simulink model "QUATERNIONS_control_law"  (R2022b)
settings: Solver=VariableStepAuto  StartTime=0.0  StopTime=10.0  RelTol=1e-3
undefined symbols (not defined in the file or in its folder): A_ATTITUDE_DET, K_d, Kp, W_e
settings Model: Creator=carlorichero  LastModifiedBy=carlorichero
settings OptimizationCC: ReuseModelBlockBuffer=on
settings RTWCC: GPUComputeCapability=5.0

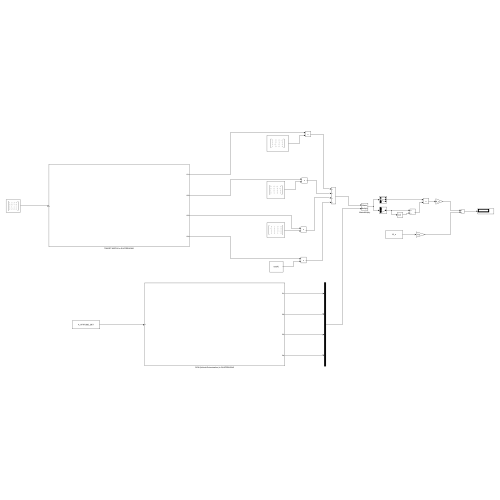
[thumbnail: Simulink's stored preview of the top-level diagram]
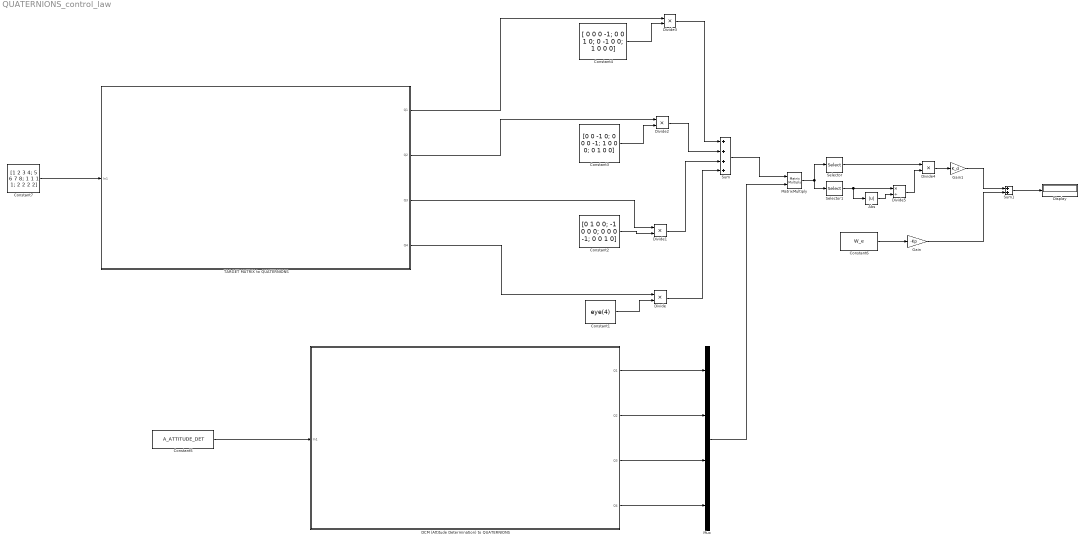
== system QUATERNIONS_control_law ==
  Abs : Abs  SaturateOnIntegerOverflow=off
  Constant1 : Constant  Value=eye(4)
  Constant2 : Constant  Value=[0 1 0 0; -1 0 0 0; 0 0 0 -1; 0 0 1 0]
  Constant3 : Constant  Value=[0 0 -1 0; 0 0 0 -1; 1 0 0 0; 0 1 0 0]
  Constant4 : Constant  Value=[ 0 0 0 -1; 0 0 1 0; 0 -1 0 0; 1 0 0 0]
  Constant5 : Constant  Value=A_ATTITUDE_DET
  Constant6 : Constant  Value=W_e
  Constant7 : Constant  Value=[1 2 3 4; 5 6 7 8; 1 1 1 1; 2 2 2 2]
  DCM (Attitude Determination) to QUATERNIONS : Subsystem
  Display : Display
  Divide{,1..4} (5 alike) : Product  Inputs=**
  Divide5 : Product  Inputs=*/
  Gain : Gain  Gain=-Kp
  Gain1 : Gain  Gain=K_d
  MatrixMultiply : Product  Multiplication=Matrix(*)
  Mux : Mux
  Selector : Selector  InputPortWidth=4  IndexOptions=Index vector (dialog)  Indices=[1 2 3]  OutputSizes=1
  Selector1 : Selector  InputPortWidth=4  IndexOptions=Index vector (dialog)  Indices=[4]  OutputSizes=1
  Sum : Sum  Inputs=++++
  Sum1 : Sum
  TARGET MATRIX to QUATERNIONS : Subsystem
  wires:
  Constant1/1 -> Divide/2
  Constant2/1 -> Divide1/2
  Constant3/1 -> Divide2/2
  Constant4/1 -> Divide3/2
  Divide3/1 -> Sum/1
  Divide2/1 -> Sum/2
  Divide1/1 -> Sum/3
  Divide/1 -> Sum/4
  Sum/1 -> MatrixMultiply/1
  Constant5/1 -> DCM (Attitude Determination) to QUATERNIONS/1(In1)
  Mux/1 -> MatrixMultiply/2
  Constant6/1 -> Gain/1
  MatrixMultiply/1 -> Selector/1, Selector1/1
  Divide4/1 -> Gain1/1
  Selector1/1 -> Abs/1, Divide5/1
  Abs/1 -> Divide5/2
  Divide5/1 -> Divide4/2
  Selector/1 -> Divide4/1
  Gain1/1 -> Sum1/1
  Gain/1 -> Sum1/2
  Sum1/1 -> Display/1
  Constant7/1 -> TARGET MATRIX to QUATERNIONS/1(In1)
  TARGET MATRIX to QUATERNIONS/1(Q1) -> Divide3/1
  TARGET MATRIX to QUATERNIONS/2(Q2) -> Divide2/1
  TARGET MATRIX to QUATERNIONS/3(Q3) -> Divide1/1
  TARGET MATRIX to QUATERNIONS/4(Q4) -> Divide/1
  DCM (Attitude Determination) to QUATERNIONS/1(Q1) -> Mux/1
  DCM (Attitude Determination) to QUATERNIONS/2(Q2) -> Mux/2
  DCM (Attitude Determination) to QUATERNIONS/3(Q3) -> Mux/3
  DCM (Attitude Determination) to QUATERNIONS/4(Q4) -> Mux/4

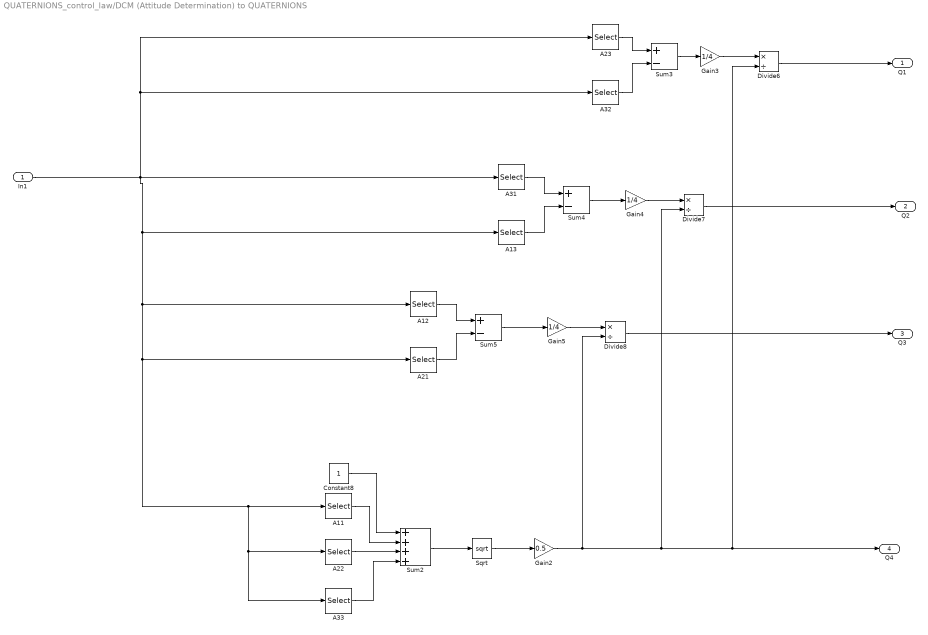
== system QUATERNIONS_control_law/DCM (Attitude Determination) to QUATERNIONS ==
  In1 : Inport
  A11 : Selector  NumberOfDimensions=2  InputPortWidth=1  IndexOptions=Index vector (dialog),Index vector (dialog)  Indices=1,1  OutputSizes=1,1
  A12 : Selector  NumberOfDimensions=2  InputPortWidth=3  IndexOptions=Index vector (dialog),Index vector (dialog)  Indices=1,2  OutputSizes=1,1
  A13 : Selector  NumberOfDimensions=2  InputPortWidth=3  IndexOptions=Index vector (dialog),Index vector (dialog)  Indices=1,3  OutputSizes=1,1
  A21 : Selector  NumberOfDimensions=2  InputPortWidth=3  IndexOptions=Index vector (dialog),Index vector (dialog)  Indices=2,1  OutputSizes=1,1
  A22 : Selector  NumberOfDimensions=2  InputPortWidth=3  IndexOptions=Index vector (dialog),Index vector (dialog)  Indices=2,2  OutputSizes=1,1
  A23 : Selector  NumberOfDimensions=2  InputPortWidth=3  IndexOptions=Index vector (dialog),Index vector (dialog)  Indices=2,3  OutputSizes=1,1
  A31 : Selector  NumberOfDimensions=2  InputPortWidth=3  IndexOptions=Index vector (dialog),Index vector (dialog)  Indices=3,1  OutputSizes=1,1
  A32 : Selector  NumberOfDimensions=2  InputPortWidth=3  IndexOptions=Index vector (dialog),Index vector (dialog)  Indices=3,2  OutputSizes=1,1
  A33 : Selector  NumberOfDimensions=2  InputPortWidth=3  IndexOptions=Index vector (dialog),Index vector (dialog)  Indices=3,3  OutputSizes=1,1
  Constant8 : Constant
  Divide6 : Product  Inputs=*/
  Divide7 : Product  Inputs=*/
  Divide8 : Product  Inputs=*/
  Gain2 : Gain  Gain=0.5
  Gain3 : Gain  Gain=1/4
  Gain4 : Gain  Gain=1/4
  Gain5 : Gain  Gain=1/4
  Sqrt : Sqrt
  Sum2 : Sum  Inputs=++++
  Sum3 : Sum  Inputs=+-
  Sum4 : Sum  Inputs=+-
  Sum5 : Sum  Inputs=+-
  Q1 : Outport
  Q2 : Outport  Port=2
  Q3 : Outport  Port=3
  Q4 : Outport  Port=4
  wires:
  Sum4/1 -> Gain4/1
  A33/1 -> Sum2/4
  Sum5/1 -> Gain5/1
  A32/1 -> Sum3/2
  Gain2/1 -> Q4/1, Divide6/2, Divide7/2, Divide8/2
  A12/1 -> Sum5/1
  Gain3/1 -> Divide6/1
  Divide8/1 -> Q3/1
  Sum2/1 -> Sqrt/1
  In1/1 -> A23/1, A32/1, A31/1, A13/1, A12/1, A21/1, A33/1, A22/1, A11/1
  Constant8/1 -> Sum2/1
  Gain5/1 -> Divide8/1
  A23/1 -> Sum3/1
  Gain4/1 -> Divide7/1
  A22/1 -> Sum2/3
  Divide6/1 -> Q1/1
  Sqrt/1 -> Gain2/1
  A11/1 -> Sum2/2
  A21/1 -> Sum5/2
  Sum3/1 -> Gain3/1
  A31/1 -> Sum4/1
  A13/1 -> Sum4/2
  Divide7/1 -> Q2/1

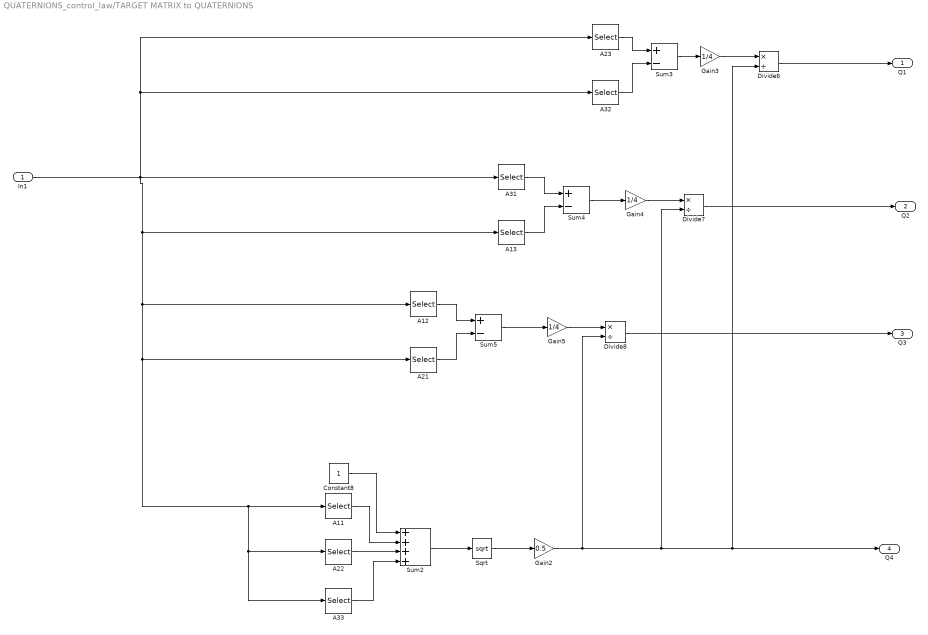
== system QUATERNIONS_control_law/TARGET MATRIX to QUATERNIONS ==
  In1 : Inport
  A11 : Selector  NumberOfDimensions=2  InputPortWidth=1  IndexOptions=Index vector (dialog),Index vector (dialog)  Indices=1,1  OutputSizes=1,1
  A12 : Selector  NumberOfDimensions=2  InputPortWidth=3  IndexOptions=Index vector (dialog),Index vector (dialog)  Indices=1,2  OutputSizes=1,1
  A13 : Selector  NumberOfDimensions=2  InputPortWidth=3  IndexOptions=Index vector (dialog),Index vector (dialog)  Indices=1,3  OutputSizes=1,1
  A21 : Selector  NumberOfDimensions=2  InputPortWidth=3  IndexOptions=Index vector (dialog),Index vector (dialog)  Indices=2,1  OutputSizes=1,1
  A22 : Selector  NumberOfDimensions=2  InputPortWidth=3  IndexOptions=Index vector (dialog),Index vector (dialog)  Indices=2,2  OutputSizes=1,1
  A23 : Selector  NumberOfDimensions=2  InputPortWidth=3  IndexOptions=Index vector (dialog),Index vector (dialog)  Indices=2,3  OutputSizes=1,1
  A31 : Selector  NumberOfDimensions=2  InputPortWidth=3  IndexOptions=Index vector (dialog),Index vector (dialog)  Indices=3,1  OutputSizes=1,1
  A32 : Selector  NumberOfDimensions=2  InputPortWidth=3  IndexOptions=Index vector (dialog),Index vector (dialog)  Indices=3,2  OutputSizes=1,1
  A33 : Selector  NumberOfDimensions=2  InputPortWidth=3  IndexOptions=Index vector (dialog),Index vector (dialog)  Indices=3,3  OutputSizes=1,1
  Constant8 : Constant
  Divide6 : Product  Inputs=*/
  Divide7 : Product  Inputs=*/
  Divide8 : Product  Inputs=*/
  Gain2 : Gain  Gain=0.5
  Gain3 : Gain  Gain=1/4
  Gain4 : Gain  Gain=1/4
  Gain5 : Gain  Gain=1/4
  Sqrt : Sqrt
  Sum2 : Sum  Inputs=++++
  Sum3 : Sum  Inputs=+-
  Sum4 : Sum  Inputs=+-
  Sum5 : Sum  Inputs=+-
  Q1 : Outport
  Q2 : Outport  Port=2
  Q3 : Outport  Port=3
  Q4 : Outport  Port=4
  wires:
  Sum4/1 -> Gain4/1
  A33/1 -> Sum2/4
  Sum5/1 -> Gain5/1
  A32/1 -> Sum3/2
  Gain2/1 -> Q4/1, Divide6/2, Divide7/2, Divide8/2
  A12/1 -> Sum5/1
  Gain3/1 -> Divide6/1
  Divide8/1 -> Q3/1
  Sum2/1 -> Sqrt/1
  In1/1 -> A23/1, A32/1, A31/1, A13/1, A12/1, A21/1, A33/1, A22/1, A11/1
  Constant8/1 -> Sum2/1
  Gain5/1 -> Divide8/1
  A23/1 -> Sum3/1
  Gain4/1 -> Divide7/1
  A22/1 -> Sum2/3
  Divide6/1 -> Q1/1
  Sqrt/1 -> Gain2/1
  A11/1 -> Sum2/2
  A21/1 -> Sum5/2
  Sum3/1 -> Gain3/1
  A31/1 -> Sum4/1
  A13/1 -> Sum4/2
  Divide7/1 -> Q2/1
